simulink model "postSNR"  (R2019a)
settings: Solver=VariableStepAuto  StartTime=0.0  StopTime=10.0  RelTol=1e-3
undefined symbols (not defined in the file or in its folder): FFT_size
settings Model: Creator=Showi  LastModifiedBy=Showi

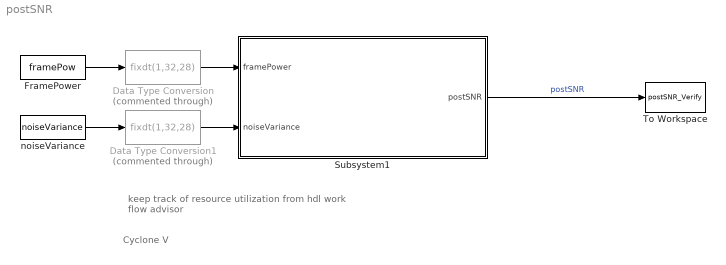
== system postSNR ==
  note: Cyclone V
  note: keep track of resource utilization from hdl work
      | flow advisor
  Data Type Conversion : DataTypeConversion  Commented=through  OutDataTypeStr=fixdt(1,32,28)
  Data Type Conversion1 : DataTypeConversion  Commented=through  OutDataTypeStr=fixdt(1,32,28)
  FramePower : FromWorkspace  VariableName=framePow  SampleTime=0
  Subsystem1 : Subsystem
  To Workspace : ToWorkspace  VariableName=postSNR_Verify  SaveFormat=Timeseries  SampleTime=-1
  noiseVariance : FromWorkspace  VariableName=noiseVariance  SampleTime=0
  wires:
  noiseVariance/1 -> Data Type Conversion1/1
  FramePower/1 -> Data Type Conversion/1
  Subsystem1/1(postSNR) -> To Workspace/1  "postSNR"
  Data Type Conversion/1 -> Subsystem1/1(framePower)
  Data Type Conversion1/1 -> Subsystem1/2(noiseVariance)

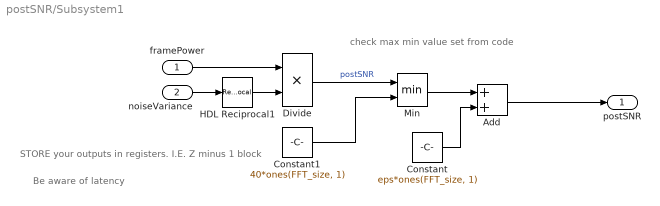
== system postSNR/Subsystem1 ==
  note: Be aware of latency
  note: STORE your outputs in registers. I.E. Z minus 1 block
  note: check max min value set from code
  framePower : Inport
  noiseVariance : Inport  Port=2
  Add : Sum
  Constant : Constant  Value=eps*ones(FFT_size, 1)  SampleTime=-1
  Constant1 : Constant  Value=40*ones(FFT_size, 1)  SampleTime=-1
  Divide : Product  Inputs=**  SaturateOnIntegerOverflow=on  RndMeth=Zero
  HDL Reciprocal1 : Reciprocal
  Min : MinMax  Inputs=2
  postSNR : Outport
  wires:
  noiseVariance/1 -> HDL Reciprocal1/1
  framePower/1 -> Divide/1
  Divide/1 -> Min/1  "postSNR"
  Constant1/1 -> Min/2
  Min/1 -> Add/1
  Add/1 -> postSNR/1
  Constant/1 -> Add/2
  HDL Reciprocal1/1 -> Divide/2
